simulink model "stm32f4_target_uart_wifi_customcode_demo"  (Simulink 7.3)
settings: Solver=ode3  SolverMode=SingleTasking  StartTime=0.0  StopTime=10.0  RelTol=1e-3
PreLoadFcn:
  | waijung.modelPreload; % Required for working with Waijung Blockset. Do not remove.
undefined symbols (not defined in the file): Data1, Data2, DestIP, DestPort, disable_rak410_setup, disable_rak410_udpsend, enable_rak410_setup, enable_rak410_udpsend, HSEOSC, in1, in2, in3, in4, Link, LQFP176, out1, output_rak410_setup, output_rak410_udpsend, Raw, ST, STM32F417IG
libraries: simulink x16, waijung_customcode x2, stm32f4_io_lib x1, stm32f4_adc_lib x1, stm32f4_device_config_lib x1
CloseFcn:
  | waijung.modelClose; % Required for working with Waijung Blockset. Do not remove.
settings Model: Creator=Krisada  LastModifiedBy=Krisada
settings OptimizationCC: OptimizeModelRefInitCode=on  LifeSpan=1
settings HardwareCC: ProdEndianess=LittleEndian  ProdHWDeviceType=ARM Compatible->Cortex - M4  TargetEndianess=LittleEndian  TargetHWDeviceType=ARM Compatible->Cortex - M4
settings RTWCC: SystemTargetFile=stm32f4.tlc  GenerateMakefile=off  TemplateMakefile=ert_default_tmf  Description=STM32F4 Target  ProcessScript=stm32f4_make_rtw_hook
settings CodeAppCC: IgnoreCustomStorageClasses=off
settings STFCustomTargetCC: ModelReferenceCompliant=off  CombineOutputUpdateFcns=on  ERTCustomFileBanners=on  SupportContinuousTime=off  SupportNonInlinedSFcns=off  SystemTargetFile=stm32f4.tlc
settings ERTTargetCC: MultiwordLength=2048  ModelReferenceCompliant=off  ParMdlRefBuildCompliant=off  CompOptLevelCompliant=off  ERTFirstTimeCompliant=off  ModelStepFunctionPrototypeControlCompliant=off  CPPClassGenCompliant=off  InlinedParameterPlacement=NonHierarchical  ERTSrcFileBannerTemplate=stm32f4_code_template.cgt  ERTHdrFileBannerTemplate=stm32f4_code_template.cgt  ERTDataSrcFileTemplate=stm32f4_code_template.cgt  ERTDataHdrFileTemplate=stm32f4_code_template.cgt  ERTCustomFileTemplate=stm32f4_file_process.tlc

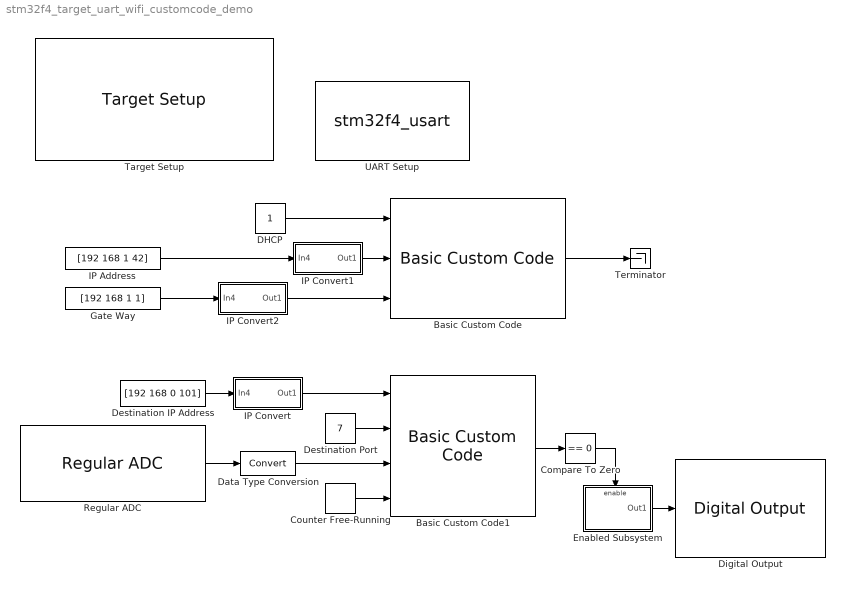
== system stm32f4_target_uart_wifi_customcode_demo ==
  Basic Custom Code : waijung_customcode/Basic Custom Code  inputporttype=uint8,uint32,uint32  cinputportlabel=DHCP,Default IP,Default Gate way  cinputportlabelstr="[\"DHCP\",\"Default IP\",\"Default Gate way\"]"  inputportcount=3  inputporttypeid="[3  7  7]"  outputporttype=uint8  coutputportlabel=Status  coutputportlabelstr="[\"Status\"]"  outputportcount=1  outputporttypeid=[3]  incpath={fullfile(pwd,'customcode_rak410')}  srcpath={fullfile(pwd,'customcode_rak410')}  incfiles={'rak410.h'}  srcfiles={'rak410.c'}  enablefuncallstr=enable_rak410_setup();  outputfuncallstr=output_rak410_setup(in1,in2,in3,out1);  disablefuncallstr=disable_rak410_setup();  sampletime=0.01  sampletimestr=0  blockid=BasicCustomCode  enablecustomportlabel=on  incfilestrarray="[\"rak410.h\"]"  inputportdiminfo="[1  1  1  3;1  1  1  7;1  1  1  7]"  outputportdiminfo="[1  1  1  3]"
  Basic Custom Code1 : waijung_customcode/Basic Custom Code  inputporttype=uint32,uint32,uint32,uint32  cinputportlabel=DestIP,DestPort,Data1,Data2  cinputportlabelstr="[\"DestIP\",\"DestPort\",\"Data1\",\"Data2\"]"  inputportcount=4  inputporttypeid="[7  7  7  7]"  outputporttype=uint8  coutputportlabel=Status  coutputportlabelstr="[\"Status\"]"  outputportcount=1  outputporttypeid=[3]  incpath={fullfile(pwd,'customcode_rak410')}  srcpath={fullfile(pwd,'customcode_rak410')}  incfiles={'rak410.h'}  srcfiles={'rak410.c'}  enablefuncallstr=enable_rak410_udpsend();  outputfuncallstr=output_rak410_udpsend(in1,in2,in3,in4,out1);  disablefuncallstr=disable_rak410_udpsend();  sampletime=-1  sampletimestr=0  blockid=BasicCustomCode1  enablecustomportlabel=on  incfilestrarray="[\"rak410.h\"]"  inputportdiminfo="[1  1  1  7;1  1  1  7;1  1  1  7;1  1  1  7]"  outputportdiminfo="[1  1  1  3]"
  Compare To Zero : simulink/Logic and Bit Operations/Compare To Zero  SystemSampleTime=-1  relop===  LogicOutDataTypeMode=uint8  ZeroCross=off
  Counter Free-Running : simulink/Sources/Counter Free-Running  SystemSampleTime=-1  NumBits=32  tsamp=-1
  DHCP : Constant  OutDataTypeMode=uint8  OutDataType=fixdt(1, 16)  OutScaling=2^0  OutDataTypeStr=uint8
  Data Type Conversion : DataTypeConversion  OutDataType=fixdt(1, 16)  OutScaling=2^0
  Destination IP Address : Constant  Value=[192 168 0 101]  OutDataTypeMode=uint32  OutDataType=fixdt(1, 16)  OutScaling=2^0  OutDataTypeStr=uint32  SampleTime=0.01
  Destination Port : Constant  Value=7  OutDataTypeMode=uint32  OutDataType=fixdt(1, 16)  OutScaling=2^0  OutDataTypeStr=uint32
  Digital Output : stm32f4_io_lib/Digital Output  use_bitband=on  port=D  speed=100  porttype=Push Pull  porttypestr=PP  use_pin0=off  use_pin1=off  use_pin2=off  use_pin3=off  use_pin4=off  use_pin5=off  use_pin6=off  use_pin7=off  use_pin8=off  use_pin9=off  use_pin10=off  use_pin11=off  use_pin12=off  use_pin13=on  use_pin14=off  use_pin15=off  pinstr=GPIO_Pin_13  usedpinarray="[0  0  0  0  0  0  0  0  0  0  0  0  0  1  0  0]"  bitbandingstr="#define DigitalOutput_D13 Peripheral_BB(GPIOD->ODR, 13)  /* Output pin */"  sampletime=-1  sampletimestr=0  blockid=DigitalOutput  enablecustomportlabel=off  globalinit=off  cinputportlabel=In1, In2  coutputportlabel=0
  Enabled Subsystem : Subsystem  TreatAsAtomicUnit=on
  Gate Way : Constant  Value=[192 168 1 1]  OutDataTypeMode=uint32  OutDataType=fixdt(1, 16)  OutScaling=2^0  OutDataTypeStr=uint32  SampleTime=0.01
  IP Address : Constant  Value=[192 168 1 42]  OutDataTypeMode=uint32  OutDataType=fixdt(1, 16)  OutScaling=2^0  OutDataTypeStr=uint32  SampleTime=0.01
  IP Convert : Subsystem
  IP Convert1 : Subsystem
  IP Convert2 : Subsystem
  Regular ADC : stm32f4_adc_lib/Regular ADC  adcmodule=1  outputdatatype=Raw (uint16)  prescaler=2  prescalerstr=ADC_Prescaler_Div2  chsamplingtime=Auto  chsamplingtimestr=ADC_SampleTime_480Cycles  read_an0=off  read_an1=off  read_an2=off  read_an3=off  read_an4=off  read_an5=on  read_an6=off  read_an7=off  read_an8=off  read_an9=off  read_an10=off  read_an11=off  read_an12=off  read_an13=off  read_an14=off  read_an15=off  read_an16=off  read_an17=off  read_an18=off  pinstr=GPIO_Pin_5  usedpinarray="[0  0  0  0  0  1  0  0  0  0  0  0  0  0  0  0  0  0  0]"  usedportidarray=[0]  usedpinidarray=[5]  usedpinidcount=1  sampletime=inf  blockid=RegularADC  enablecustomportlabel=off  cinputportlabel=0  coutputportlabel=Out1, Out2
  Target Setup : stm32f4_device_config_lib/Target Setup  Priority=100  compiler=GNU ARM  previous_compiler=GNU ARM  mcu=STM32F417IG (LQFP176)  mcustr=STM32F417IG  clockconfig=HSEOSC-8MHz  system_stm32f4xx_c_path=F:\trunk\targets\stm32f4_target\stm32f4\utils\system_stm32f4xx_default\STM32F40_41xxx\hseosc8mhz  showmemoryconfiguration=off  stacksize=0x2000  heapsize=0x2000  enableautocompiledownload=on  fullchiperase=off  programmerinterface=ST-Link  editctrlstr=on  compilercontrolstr=$(patsubst %, -I%, .) -mcpu=cortex-m4 -mthumb -mthumb-interwork -mfloat-abi=hard -mfpu=fpv4-sp-d16 -ffast-math -Wall -Wextra -Ofast  assemblercontrolstr=$(patsubst %, -I%, .) -mcpu=cortex-m4 -mthumb -mthumb-interwork -mfloat-abi=hard -mfpu=fpv4-sp-d16 -ffast-math -Wall -Wextra -Ofast -Wa,-amhls=$(<:.s=.lst) -D__STACK_SIZE=$(STACK_SIZE) -D__HEAP_SIZE=$(HEAP_SIZE)  linkercontrolstr=-T$(LD_SCRIPT) -g -Wl,-Map=$(MAP),--cref,--no-warn-mismatch -mcpu=cortex-m4 -mthumb -mthumb-interwork -mfloat-abi=hard -mfpu=fpv4-sp-d16 -specs=nosys.specs  runafterdownload=on  execprofile=None  profileruart=3  profilerbaud=500000  profilertxpin=D8  profilerinitstr=0.01,168000000,1680000,500000,0  manualsetsampletime=off  sampletime=0.01  blockid=TargetSetup  systickreloadvalue=1680000  hseval=8000000  lastprofileruart=3  hclk=168000000  flashorigin=0x8000000  flashlength=1024k  ramorigin=0x20000000  ramlength=128k  useextram=off
  Terminator : Terminator
  UART Setup : S-Function  Priority=1  FunctionName=stm32f4_usart  Parameters=configuration,uartmodule,transfer,baudrate,inputtype,outputtype,confstr,binheaderarray,binterminatorarray,asciiheader,asciiterminator,bindatalength,packetmode,varname,sampletime,sampletimestr,blockid  EnableBusSupport=off  mask(stm32f4_usart){configuration=Setup, uartmodule=2, baudrate=115200, databits=8, parity=No, stopbit=1, remaptxpin=A2, remaprxpin=A3, flowcontrol=RTS/CTS, remapctspin=A0, remaprtspin=A1, advanceoptions=on, rxbuffersize=512, txbuffersize=512, transfer=Blocking, packetmode=Ascii, binheader='7E 7E', binterminator='03 03', porttype_double=1, porttype_single=0, porttype_int8=1, porttype_uint8=0, porttype_int16=0, porttype_uint16=0, porttype_int32=0, porttype_uint32=0, asciiformat='%d,%f', rx_asciiterminator=CRLF (0x0D 0x0A - "\r\n"), tx_asciiterminator=CR (0x0D - "\r"), storagename=<empty>, varname=, inputtype=[0], outputtype=[0], binheaderarray=[0], binterminatorarray=[0], bindatalength=0, asciiheader='', asciiterminator=[0], sampletime=-1, sampletimestr=0, blockid=UARTSetup, confstr=[ "dummy", "1", "A", "2", "1", "A", "3", "1", "A", "0", "1", "A", "1", "1", "4", "6", "1", "4", "5", "512", "512", "1", "2", "115200", "8", "No", "1", "RTS_CTS", "USART2"], lastmodule=2}
      mask prompts: uartmodule "UART Module"; baudrate "Baud rate (bps)"; databits "Data bits"; stopbit "Stop bit"; remaptxpin "Tx Pin"; remaprxpin "Rx Pin"; flowcontrol "Hardware flow control"; remapctspin "HW Flow control, CTS Pin"; remaprtspin "HW Flow control, RTS Pin"; advanceoptions "Advance options"; rxbuffersize "Rx buffer size (bytes)"; txbuffersize "Tx buffer size (bytes)"; packetmode "Packet mode"; binheader "Binary header (example: '7E 7E')"; binterminator "Binary terminator (example: '03 03')"; porttype_double "Number of data port, type DOUBLE"; porttype_single "Number of data port, type SINGLE"; porttype_int8 "Number of data port, type INT8"; porttype_uint8 "Number of data port, type UINT8"; porttype_int16 "Number of data port, type INT16"; porttype_uint16 "Number of data port, type UINT16"; porttype_int32 "Number of data port, type INT32"; porttype_uint32 "Number of data port, type UINT32"; asciiformat "Ascii format"; rx_asciiterminator "End of packet"; tx_asciiterminator "End of packet"; storagename "Buffer"; varname "Var name"; inputtype "Input data type"; outputtype "Output data type"; binheaderarray "Binary header"; binterminatorarray "Binary terminator"; bindatalength "Binary data length"; asciiheader "Ascii header (printf format)"; asciiterminator "Ascii terminator"; sampletime "Sample time (sec)"; sampletimestr "Compiled sample time (sec) in string"; confstr "Configuration string"; lastmodule "Last module selected"
      mask help:
      | Default STM32F4DISCOVERY + aMG F4 Connect 2 + aMG USB Converter N2 settings use
      |
      | USART3, Tx D8, Rx D9 and USB Serial Converter A.
      mask init:
      | stm32f4_usart_callback('init');
      mask Help: web(fullfile(waijungdocroot,'stm32f4_usart_setup.htm'), '-browser')
      mask StyleString: popup(Setup|Tx|Rx),popup(1|2|3|4|5|6),edit,popup(8),popup(No|Odd|Even),popup(0.5|1|1.5|2),popup(Not used|A2|D5),popup(Not used|A3|D6),popup(None|RTS|CTS|RTS/CTS),popup(Not used|A0|D3),popup(Not used|A1|D4),checkbox,popup(16|32|64|128|256|512|1024|2048),popup(16|32|64|128|256|512|1024|2048),popup(Blocking|Non-Blocking),popup(Ascii|Binary|String Buffer),edit,edit,edit,edit,edit,edit,edit,edit,edit,edit,edit,popup(CR (0x0D - "\r")|LF (0x0A - "\n")|CRLF (0x0D 0x0A - "\r\n")),popup(CR (0x0D - "\r")|LF (0x0A - "\n")|CRLF (0x0D 0x0A - "\r\n")|None),popup(<empty>),edit,edit,edit,edit,edit,edit,edit,edit,edit,edit,edit,edit,edit
      mask CallbackString: stm32f4_usart_callback('configuration');|stm32f4_usart_callback('uartmodule');|stm32f4_usart_callback('baudrate');||||||stm32f4_usart_callback('flowcontrol');|||stm32f4_usart_callback('advanceoptions');|||stm32f4_usart_callback('transfer');|stm32f4_usart_callback('packetmode');|stm32f4_usart_callback('binheader');|stm32f4_usart_callback('binterminator');|stm32f4_usart_callback('porttype');|stm32f4_usart_callback('porttype');|stm32f4_usart_callback('porttype');|stm32f4_usart_callback('porttype');|stm32f4_usart_callback('porttype');|stm32f4_usart_callback('porttype');|stm32f4_usart_callback('porttype');|stm32f4_usart_callback('porttype');|stm32f4_usart_callback('asciiformat');|stm32f4_usart_callback('rx_asciiterminator');|stm32f4_usart_callback('tx_asciiterminator');|stm32f4_usart_callback('storagename');|stm32f4_usart_callback('varname');||||||||stm32f4_usart_callback('sampletime');|stm32f4_usart_callback('sampletimestr');|stm32f4_usart_callback('blockid');||
      mask Display: text(0.5, 0.5, 'Module: USART2_Setup\nBaud (Bps): 115200\nDMA Buffer: 512/512\nTx/Rx Pin: A2/A3\nCts/Rts Pin: A0/A1','ver','middle','hor','center');
  wires:
  Destination IP Address/1 -> IP Convert/1(In4)
  Basic Custom Code1/1 -> Compare To Zero/1
  IP Convert/1(Out1) -> Basic Custom Code1/1
  Destination Port/1 -> Basic Custom Code1/2
  Regular ADC/1 -> Data Type Conversion/1
  Compare To Zero/1 -> Enabled Subsystem/Enable
  Enabled Subsystem/1(Out1) -> Digital Output/1
  DHCP/1 -> Basic Custom Code/1
  IP Convert1/1(Out1) -> Basic Custom Code/2
  IP Convert2/1(Out1) -> Basic Custom Code/3
  IP Address/1 -> IP Convert1/1(In4)
  Gate Way/1 -> IP Convert2/1(In4)
  Data Type Conversion/1 -> Basic Custom Code1/3
  Counter Free-Running/1 -> Basic Custom Code1/4
  Basic Custom Code/1 -> Terminator/1

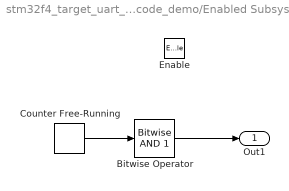
== system stm32f4_target_uart_wifi_customcode_demo/Enabled Subsystem ==
  Enable : EnablePort
  Bitwise Operator : simulink/Logic and Bit Operations/Bitwise Operator  logicop=AND  UseBitMask=on  BitMask=1  BitMaskRealWorld=Stored Integer
  Counter Free-Running : simulink/Sources/Counter Free-Running  SystemSampleTime=-1  NumBits=16  tsamp=-1
  Out1 : Outport  OutDataType=fixdt(1, 16)  OutScaling=2^0
  wires:
  Counter Free-Running/1 -> Bitwise Operator/1
  Bitwise Operator/1 -> Out1/1

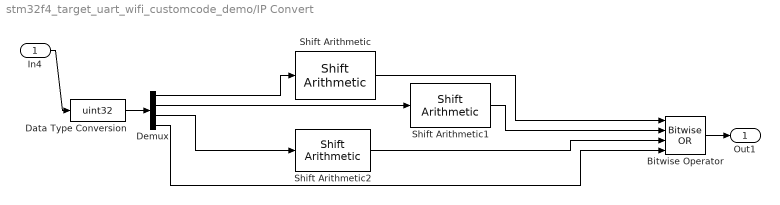
== system stm32f4_target_uart_wifi_customcode_demo/IP Convert ==
  In4 : Inport
  Bitwise Operator : simulink/Logic and Bit Operations/Bitwise Operator  logicop=OR  UseBitMask=off  NumInputPorts=4  BitMask=bin2dec('11011001')  BitMaskRealWorld=Stored Integer
  Data Type Conversion : DataTypeConversion  OutDataTypeMode=uint32  OutDataType=fixdt(1, 16)  OutScaling=2^0  OutDataTypeStr=uint32
  Demux : Demux
  Shift Arithmetic : simulink/Logic and Bit Operations/Shift Arithmetic  SystemSampleTime=-1  nBitShiftRight=-24  nBinPtShiftRight=0
  Shift Arithmetic1 : simulink/Logic and Bit Operations/Shift Arithmetic  SystemSampleTime=-1  nBitShiftRight=-16  nBinPtShiftRight=0
  Shift Arithmetic2 : simulink/Logic and Bit Operations/Shift Arithmetic  SystemSampleTime=-1  nBitShiftRight=-8  nBinPtShiftRight=0
  Out1 : Outport
  wires:
  Demux/4 -> Bitwise Operator/4
  Demux/3 -> Shift Arithmetic2/1
  In4/1 -> Data Type Conversion/1
  Bitwise Operator/1 -> Out1/1
  Demux/2 -> Shift Arithmetic1/1
  Demux/1 -> Shift Arithmetic/1
  Shift Arithmetic2/1 -> Bitwise Operator/3
  Shift Arithmetic1/1 -> Bitwise Operator/2
  Shift Arithmetic/1 -> Bitwise Operator/1
  Data Type Conversion/1 -> Demux/1

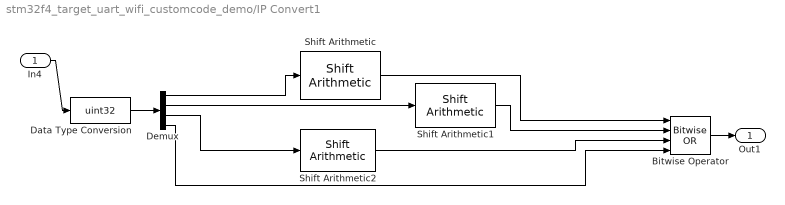
== system stm32f4_target_uart_wifi_customcode_demo/IP Convert1 ==
  In4 : Inport
  Bitwise Operator : simulink/Logic and Bit Operations/Bitwise Operator  logicop=OR  UseBitMask=off  NumInputPorts=4  BitMask=bin2dec('11011001')  BitMaskRealWorld=Stored Integer
  Data Type Conversion : DataTypeConversion  OutDataTypeMode=uint32  OutDataType=fixdt(1, 16)  OutScaling=2^0  OutDataTypeStr=uint32
  Demux : Demux
  Shift Arithmetic : simulink/Logic and Bit Operations/Shift Arithmetic  SystemSampleTime=-1  nBitShiftRight=-24  nBinPtShiftRight=0
  Shift Arithmetic1 : simulink/Logic and Bit Operations/Shift Arithmetic  SystemSampleTime=-1  nBitShiftRight=-16  nBinPtShiftRight=0
  Shift Arithmetic2 : simulink/Logic and Bit Operations/Shift Arithmetic  SystemSampleTime=-1  nBitShiftRight=-8  nBinPtShiftRight=0
  Out1 : Outport
  wires:
  Shift Arithmetic/1 -> Bitwise Operator/1
  Shift Arithmetic1/1 -> Bitwise Operator/2
  Shift Arithmetic2/1 -> Bitwise Operator/3
  Demux/1 -> Shift Arithmetic/1
  Demux/2 -> Shift Arithmetic1/1
  Bitwise Operator/1 -> Out1/1
  In4/1 -> Data Type Conversion/1
  Demux/3 -> Shift Arithmetic2/1
  Demux/4 -> Bitwise Operator/4
  Data Type Conversion/1 -> Demux/1

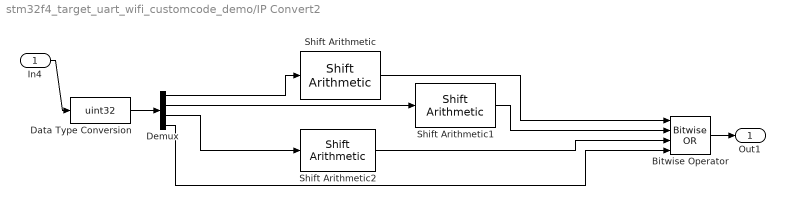
== system stm32f4_target_uart_wifi_customcode_demo/IP Convert2 ==
  In4 : Inport
  Bitwise Operator : simulink/Logic and Bit Operations/Bitwise Operator  logicop=OR  UseBitMask=off  NumInputPorts=4  BitMask=bin2dec('11011001')  BitMaskRealWorld=Stored Integer
  Data Type Conversion : DataTypeConversion  OutDataTypeMode=uint32  OutDataType=fixdt(1, 16)  OutScaling=2^0  OutDataTypeStr=uint32
  Demux : Demux
  Shift Arithmetic : simulink/Logic and Bit Operations/Shift Arithmetic  SystemSampleTime=-1  nBitShiftRight=-24  nBinPtShiftRight=0
  Shift Arithmetic1 : simulink/Logic and Bit Operations/Shift Arithmetic  SystemSampleTime=-1  nBitShiftRight=-16  nBinPtShiftRight=0
  Shift Arithmetic2 : simulink/Logic and Bit Operations/Shift Arithmetic  SystemSampleTime=-1  nBitShiftRight=-8  nBinPtShiftRight=0
  Out1 : Outport
  wires:
  Data Type Conversion/1 -> Demux/1
  Demux/4 -> Bitwise Operator/4
  Demux/3 -> Shift Arithmetic2/1
  In4/1 -> Data Type Conversion/1
  Bitwise Operator/1 -> Out1/1
  Demux/2 -> Shift Arithmetic1/1
  Demux/1 -> Shift Arithmetic/1
  Shift Arithmetic2/1 -> Bitwise Operator/3
  Shift Arithmetic1/1 -> Bitwise Operator/2
  Shift Arithmetic/1 -> Bitwise Operator/1
